simulink model "ObservadorControlInteligente"  (R2017b)
settings: Solver=VariableStepAuto  StartTime=0.0  StopTime=10.0  RelTol=1e-3
undefined symbols (not defined in the file): g, k, l, L1, L2, ml
settings Model: Creator=Benjamin Nicolas  LastModifiedBy=Benjamin Nicolas

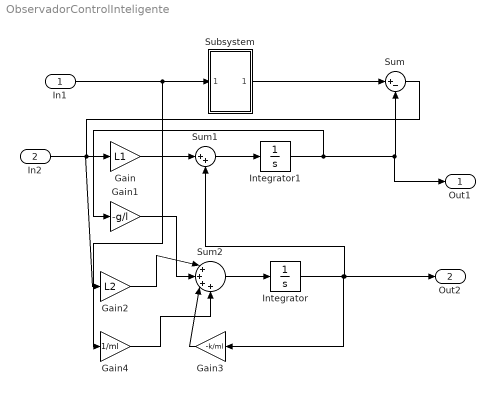
== system ObservadorControlInteligente ==
  In1 : Inport
  In2 : Inport  Port=2
  Gain : Gain  Gain=L1
  Gain1 : Gain  Gain=-g/l
  Gain2 : Gain  Gain=L2
  Gain3 : Gain  Gain=-k/ml
  Gain4 : Gain  Gain=1/ml
  Integrator : Integrator
  Integrator1 : Integrator
  Subsystem : Subsystem
  Sum : Sum  Inputs=|+-
  Sum1 : Sum  Inputs=|++
  Sum2 : Sum  Inputs=|++++
  Out1 : Outport
  Out2 : Outport  Port=2
  wires:
  In1/1 -> Gain4/1, Subsystem/1(In1)
  Subsystem/1(Out1) -> Sum/1
  Gain/1 -> Sum1/1
  Sum2/1 -> Integrator/1
  Integrator/1 -> Out2/1, Sum1/2, Gain3/1
  Sum1/1 -> Integrator1/1
  Integrator1/1 -> Gain1/1, Out1/1, Sum/2
  Sum/1 -> Gain2/1, Gain/1
  Gain2/1 -> Sum2/1
  Gain1/1 -> Sum2/2
  Gain3/1 -> Sum2/3
  Gain4/1 -> Sum2/4
  In2/1 -> ?

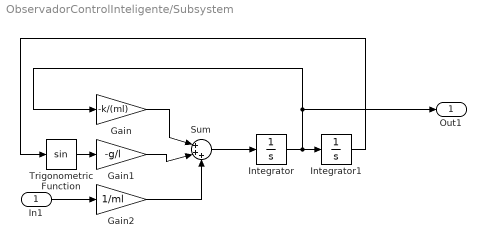
== system ObservadorControlInteligente/Subsystem ==
  In1 : Inport
  Gain : Gain  Gain=-k/(ml)
  Gain1 : Gain  Gain=-g/l
  Gain2 : Gain  Gain=1/ml
  Integrator : Integrator
  Integrator1 : Integrator
  Sum : Sum  Inputs=|+++
  Trigonometric Function : Trigonometry
  Out1 : Outport
  wires:
  Gain/1 -> Sum/1
  Integrator1/1 -> Trigonometric Function/1
  Trigonometric Function/1 -> Gain1/1
  In1/1 -> Gain2/1
  Integrator/1 -> Out1/1, Gain/1, Integrator1/1
  Sum/1 -> Integrator/1
  Gain1/1 -> Sum/2
  Gain2/1 -> Sum/3
